simulink model "sl_subsys_trig3"  (Simulink 6.0)
settings: Solver=FixedStepDiscrete  StartTime=0.0  StopTime=10.0  RelTol=1e-3
settings Model: CovMetricSettings=d  Creator=The MathWorks Inc.  LastModifiedBy=batserve  ExtModeAutoUpdateStatusClock=off
settings OptimizationCC: BlockReduction=off  BooleanDataType=off
settings DebuggingCC: CheckExecutionContextPreStartOutputMsg=on  CheckExecutionContextRuntimeOutputMsg=on  SolverPrmCheckMsg=none
settings HardwareCC: TargetUnknown=on

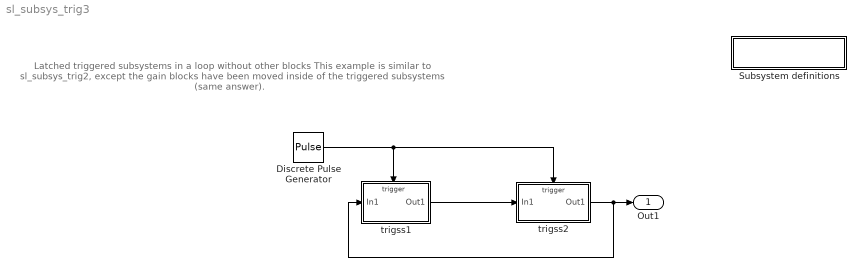
== system sl_subsys_trig3 ==
  note: Latched triggered subsystems in a loop without other blocks
      |
      | This example is similar to sl_subsys_trig2, except the gain blocks
      | have been moved inside of the triggered subsystems (same answer).
  " Subsystem definitions" : Subsystem  PropExecContextAcrossSSBoundary=on
      settings: OpenFcn=helpview([matlabroot,'/toolbox/simulink/simdemos/sl_subsys_definitions.html']);
      mask Display: disp('Subsystem\ndefinitions')
  Discrete Pulse Generator : DiscretePulseGenerator
  trigss1 : Subsystem  TreatAsAtomicUnit=on  PropExecContextAcrossSSBoundary=on
  trigss2 : Subsystem  TreatAsAtomicUnit=on  PropExecContextAcrossSSBoundary=on
  Out1 : Outport
  wires:
  trigss1/1(Out1) -> trigss2/1(In1)
  trigss2/1(Out1) -> Out1/1, trigss1/1(In1)
  Discrete Pulse Generator/1 -> trigss1/Trigger, trigss2/Trigger

== system sl_subsys_trig3/ Subsystem definitions ==

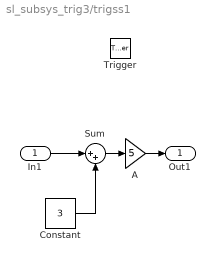
== system sl_subsys_trig3/trigss1 ==
  In1 : Inport  Port=1  LatchInput=on
  Trigger : TriggerPort
  A : Gain  Gain=5  SaturateOnIntegerOverflow=on
  Constant : Constant  Value=3
  Sum : Sum  Inputs=|++  SaturateOnIntegerOverflow=on  InputSameDT=on
  Out1 : Outport
  wires:
  In1/1 -> Sum/1
  Sum/1 -> A/1
  Constant/1 -> Sum/2
  A/1 -> Out1/1

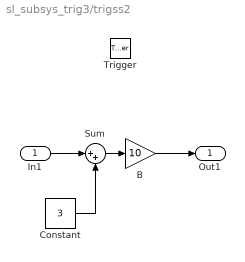
== system sl_subsys_trig3/trigss2 ==
  In1 : Inport  Port=1  LatchInput=on
  Trigger : TriggerPort
  B : Gain  Gain=10  SaturateOnIntegerOverflow=on
  Constant : Constant  Value=3
  Sum : Sum  Inputs=|++  SaturateOnIntegerOverflow=on  InputSameDT=on
  Out1 : Outport
  wires:
  Constant/1 -> Sum/2
  Sum/1 -> B/1
  In1/1 -> Sum/1
  B/1 -> Out1/1
